simulink model "BattTest"  (Simulink 4.00)
settings: Solver=ode5  StartTime=0.0  StopTime=1  FixedStep=0.01  RelTol=1e-3
values from neighbouring files (symbols this model uses):
  SOC_beg = 70    [AGM_ini_file.m]    (also in DP_Batt_Init.m = battery.init_SOC)
undefined symbols (not defined in the file or in its folder): battery
libraries: simulink3 x6
settings Model: LastModifiedBy=Mark

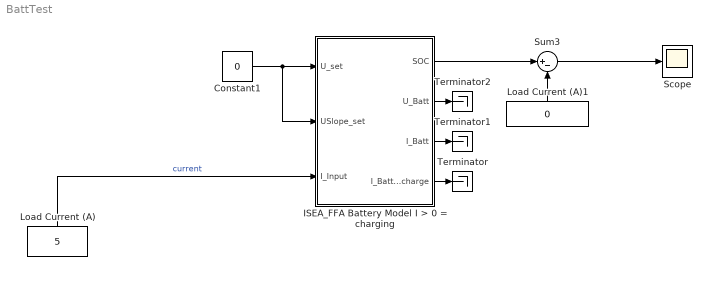
== system BattTest ==
  Constant1 : Constant  Value=0
  ISEA_FFA Battery Model I > 0 = charging : Subsystem
      settings: RTWFcnNameOpts=Auto  RTWFileNameOpts=Auto
  Load Current (A) : Constant  Orientation=up  Value=5
  Load Current (A)1 : Constant  Orientation=up  Value=0
  Scope : Scope
      settings: TimeRange=auto  YMin=-5  YMax=5  SaveToWorkspace=off  SaveName=ScopeData  LimitDataPoints=on  MaxDataPoints=5000
  Sum3 : Sum  Inputs=|+-  SaturateOnIntegerOverflow=on
  Terminator : Terminator
  Terminator1 : Terminator
  Terminator2 : Terminator
  wires:
  Sum3/1 -> Scope/1
  Load Current (A)1/1 -> Sum3/2
  Constant1/1 -> ISEA_FFA Battery Model I > 0 = charging/1(U_set), ISEA_FFA Battery Model I > 0 = charging/2(USlope_set)
  ISEA_FFA Battery Model I > 0 = charging/1(SOC) -> Sum3/1
  ISEA_FFA Battery Model I > 0 = charging/2(U_Batt) -> Terminator2/1
  ISEA_FFA Battery Model I > 0 = charging/3(I_Batt) -> Terminator1/1
  ISEA_FFA Battery Model I > 0 = charging/4(I_Batt_max_charge) -> Terminator/1
  Load Current (A)/1 -> ISEA_FFA Battery Model I > 0 = charging/3(I_Input)  "current"

== system BattTest/ISEA_FFA Battery Model I > 0 = charging ==
  U_set : Inport  Port=1  LatchInput=off
  USlope_set : Inport  Port=2  LatchInput=off
  I_Input : Inport  Port=3  LatchInput=off
  Batterie : Subsystem
      settings: RTWFcnNameOpts=Auto  RTWFileNameOpts=Auto
  Mux : Mux  Inputs=2
  initial battery SOC : Constant  Value=SOC_beg
  SOC : Outport  Port=1
  U_Batt : Outport  Port=2
  I_Batt : Outport  Port=3
  I_Batt_max_charge : Outport  Port=4
  wires:
  Batterie/4(SOC) -> SOC/1
  Batterie/3(BUS_U_out) -> U_Batt/1  "BUS_U"
  Mux/1 -> Batterie/1(BUS_1_in1)  "BUS_1"
  initial battery SOC/1 -> Mux/2  "SOC_beg"
  I_Input/1 -> Mux/1
  Batterie/2(I_Batt) -> I_Batt/1
  U_set/1 -> Batterie/2(U_set)
  Batterie/1(I_Batt_max_charge) -> I_Batt_max_charge/1
  USlope_set/1 -> Batterie/3(USlope_set)

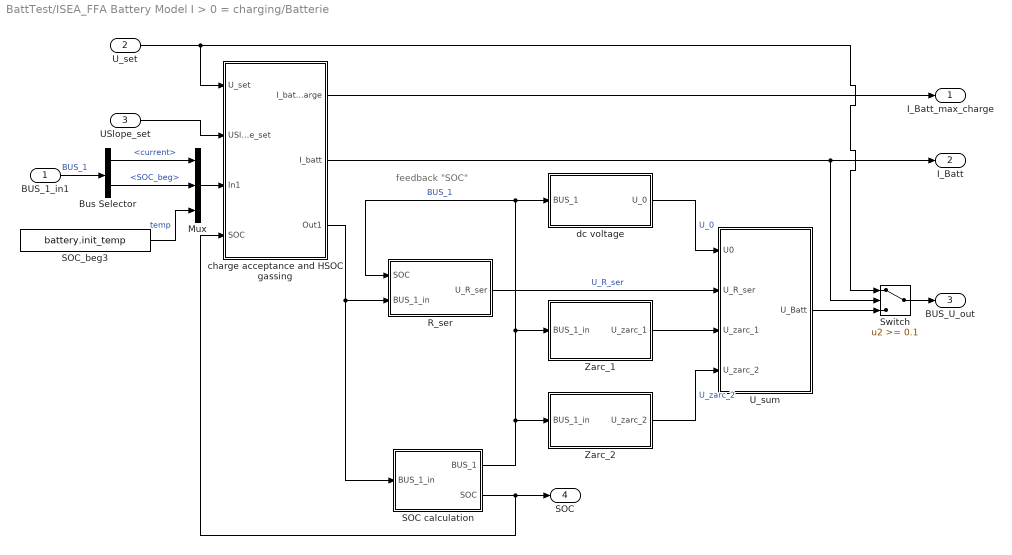
== system BattTest/ISEA_FFA Battery Model I > 0 = charging/Batterie ==
  note: feedback "SOC"
  BUS_1_in1 : Inport  Port=1  LatchInput=off
  U_set : Inport  Port=2  LatchInput=off
  USlope_set : Inport  Port=3  LatchInput=off
  Bus Selector : BusSelector  OutputSignals=current,SOC_beg  MuxedOutput=off
  Mux : Mux  Inputs=3
  R_ser : Subsystem
      settings: RTWFcnNameOpts=Auto  RTWFileNameOpts=Auto
  SOC calculation : Subsystem
      settings: RTWFcnNameOpts=Auto  RTWFileNameOpts=Auto
  SOC_beg3 : Constant  Value=battery.init_temp
  Switch : Switch  Threshold=0.1
  U_sum : Subsystem
      settings: RTWFcnNameOpts=Auto  RTWFileNameOpts=Auto
  Zarc_1 : Subsystem
      settings: RTWFcnNameOpts=Auto  RTWFileNameOpts=Auto
  Zarc_2 : Subsystem
      settings: RTWFcnNameOpts=Auto  RTWFileNameOpts=Auto
  charge acceptance and HSOC gassing : Subsystem
      settings: RTWFcnNameOpts=Auto  RTWFileNameOpts=Auto
  dc voltage : Subsystem
      settings: RTWFcnNameOpts=Auto  RTWFileNameOpts=Auto
  I_Batt_max_charge : Outport  Port=1
  I_Batt : Outport  Port=2
  BUS_U_out : Outport  Port=3
  SOC : Outport  Port=4
  wires:
  SOC calculation/2(SOC) -> SOC/1, charge acceptance and HSOC gassing/4(SOC)
  SOC_beg3/1 -> Mux/3  "temp"
  BUS_1_in1/1 -> Bus Selector/1  "BUS_1"
  Mux/1 -> charge acceptance and HSOC gassing/3(In1)
  Bus Selector/2 -> Mux/2  "<SOC_beg>"
  Bus Selector/1 -> Mux/1  "<current>"
  Zarc_1/1(U_zarc_1) -> U_sum/3(U_zarc_1)
  Zarc_2/1(U_zarc_2) -> U_sum/4(U_zarc_2)  "U_zarc_2"
  SOC calculation/1(BUS_1) -> Zarc_2/1(BUS_1_in), dc voltage/1(BUS_1), R_ser/1(SOC), Zarc_1/1(BUS_1_in)  "BUS_1"
  dc voltage/1(U_0) -> U_sum/1(U0)  "U_0"
  R_ser/1(U_R_ser) -> U_sum/2(U_R_ser)  "U_R_ser"
  charge acceptance and HSOC gassing/3(Out1) -> R_ser/2(BUS_1_in), SOC calculation/1(BUS_1_in)
  U_sum/1(U_Batt) -> Switch/3
  Switch/1 -> BUS_U_out/1
  charge acceptance and HSOC gassing/2(I_batt) -> I_Batt/1, Switch/2
  charge acceptance and HSOC gassing/1(I_bat_max_charge) -> I_Batt_max_charge/1
  USlope_set/1 -> charge acceptance and HSOC gassing/2(USlope_set)
  U_set/1 -> charge acceptance and HSOC gassing/1(U_set), Switch/1

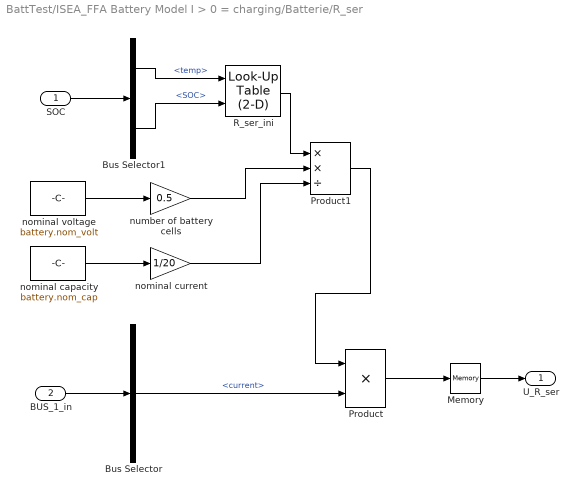
== system BattTest/ISEA_FFA Battery Model I > 0 = charging/Batterie/R_ser ==
  SOC : Inport  Port=1  LatchInput=off
  BUS_1_in : Inport  Port=2  LatchInput=off
  Bus Selector : BusSelector  OutputSignals=current  MuxedOutput=off
  Bus Selector1 : BusSelector  OutputSignals=temp,SOC  MuxedOutput=off
  Memory : Memory  X0=0  InheritSampleTime=off
      settings: RTWStateStorageClass=Auto
  Product : Product  Inputs=2  Multiplication=Element-wise(.*)  SaturateOnIntegerOverflow=on
  Product1 : Product  Inputs=**/  Multiplication=Element-wise(.*)  SaturateOnIntegerOverflow=on
  R_ser_ini : simulink3/Functions & Tables/Look-Up Table (2-D)  x=battery.temp_in  y=battery.SOC_in  t=battery.R_ser_ini
  nominal capacity : Constant  Value=battery.nom_cap
  nominal current : Gain  Gain=1/20  Multiplication=Element-wise(K.*u)  SaturateOnIntegerOverflow=on
  nominal voltage : Constant  Value=battery.nom_volt
  number of battery cells : Gain  Gain=0.5  Multiplication=Element-wise(K.*u)  SaturateOnIntegerOverflow=on
  U_R_ser : Outport  Port=1
  wires:
  Memory/1 -> U_R_ser/1
  nominal capacity/1 -> nominal current/1
  nominal current/1 -> Product1/3
  Product1/1 -> Product/1
  number of battery cells/1 -> Product1/2
  nominal voltage/1 -> number of battery cells/1
  R_ser_ini/1 -> Product1/1
  Bus Selector1/1 -> R_ser_ini/1  "<temp>"
  Bus Selector1/2 -> R_ser_ini/2  "<SOC>"
  SOC/1 -> Bus Selector1/1
  Product/1 -> Memory/1
  Bus Selector/1 -> Product/2  "<current>"
  BUS_1_in/1 -> Bus Selector/1

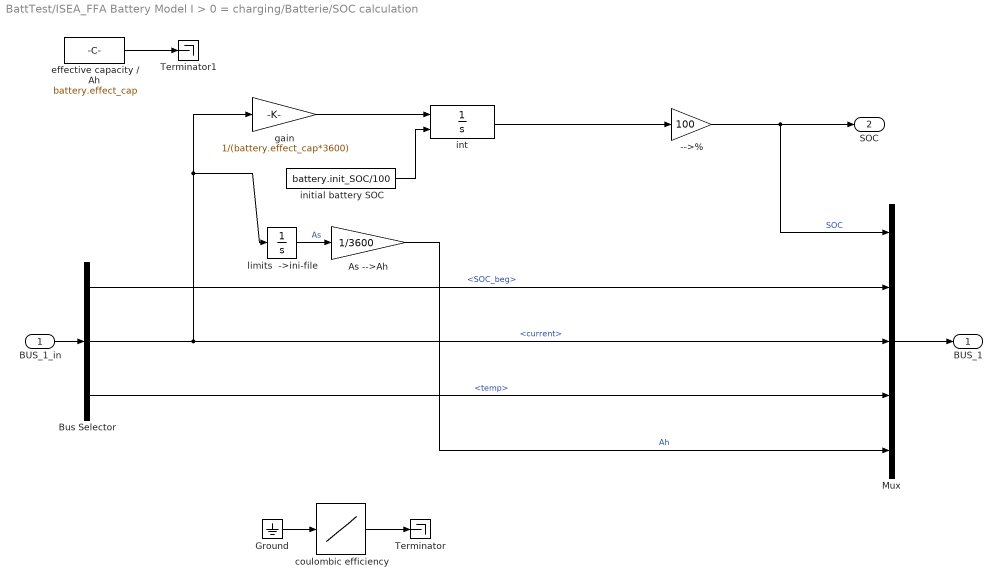
== system BattTest/ISEA_FFA Battery Model I > 0 = charging/Batterie/SOC calculation ==
  BUS_1_in : Inport  Port=1  LatchInput=off
  -->% : Gain  Gain=100  Multiplication=Element-wise(K.*u)  SaturateOnIntegerOverflow=on
  As -->Ah : Gain  Gain=1/3600  Multiplication=Element-wise(K.*u)  SaturateOnIntegerOverflow=on
  Bus Selector : BusSelector  OutputSignals=SOC_beg,current,temp  MuxedOutput=off
  Ground : Ground
  Mux : Mux  Inputs=5
  Terminator : Terminator
  Terminator1 : Terminator
  coulombic efficiency : Lookup  InputValues=[-1 0 1]  OutputValues=[-1 0 battery.eta_coulomb/100]
  "effective capacity / Ah " : Constant  Value=battery.effect_cap
  gain : Gain  Gain=1/(battery.effect_cap*3600)  Multiplication=Element-wise(K.*u)  SaturateOnIntegerOverflow=on
  initial battery SOC : Constant  Value=battery.init_SOC/100
  int : Integrator  ExternalReset=none  InitialConditionSource=external  InitialCondition=0  LimitOutput=on  UpperSaturationLimit=1  LowerSaturationLimit=0  ShowSaturationPort=off  ShowStatePort=off  AbsoluteTolerance=auto
  limits  ->ini-file : Integrator  ExternalReset=none  InitialConditionSource=internal  InitialCondition=0  LimitOutput=on  UpperSaturationLimit=battery.up_lim_soc_calc  LowerSaturationLimit=battery.low_lim_soc_calc  ShowSaturationPort=off  ShowStatePort=off  AbsoluteTolerance=auto
  BUS_1 : Outport  Port=1
  SOC : Outport  Port=2
  wires:
  -->%/1 -> Mux/1, SOC/1  "SOC"
  int/1 -> -->%/1
  As -->Ah/1 -> Mux/5  "Ah"
  limits  ->ini-file/1 -> As -->Ah/1  "As"
  Bus Selector/1 -> Mux/2  "<SOC_beg>"
  Bus Selector/2 -> Mux/3, limits  ->ini-file/1, gain/1  "<current>"
  Mux/1 -> BUS_1/1
  Bus Selector/3 -> Mux/4  "<temp>"
  BUS_1_in/1 -> Bus Selector/1
  Ground/1 -> coulombic efficiency/1
  coulombic efficiency/1 -> Terminator/1
  initial battery SOC/1 -> int/2
  gain/1 -> int/1
  "effective capacity / Ah "/1 -> Terminator1/1

== system BattTest/ISEA_FFA Battery Model I > 0 = charging/Batterie/U_sum ==
  U0 : Inport  Port=1  LatchInput=off
  U_R_ser : Inport  Port=2  LatchInput=off
  U_zarc_1 : Inport  Port=3  LatchInput=off
  U_zarc_2 : Inport  Port=4  LatchInput=off
  Bus Selector2 : BusSelector  OutputSignals=U_2c,U_2b,U_2d  MuxedOutput=off
  Sum : Sum  Inputs=+++++  SaturateOnIntegerOverflow=on
  Sum3 : Sum  Inputs=+++  SaturateOnIntegerOverflow=on
  U_L : Constant  Value=0
  U_Batt : Outport  Port=1
  wires:
  U_L/1 -> Sum/2
  U_zarc_1/1 -> Sum/4
  U_zarc_2/1 -> Bus Selector2/1
  Sum3/1 -> Sum/5
  U0/1 -> Sum/1
  Bus Selector2/3 -> Sum3/3  "<U_2d>"
  Bus Selector2/2 -> Sum3/2  "<U_2b>"
  Bus Selector2/1 -> Sum3/1  "<U_2c>"
  Sum/1 -> U_Batt/1  "U_ges"
  U_R_ser/1 -> Sum/3

== system BattTest/ISEA_FFA Battery Model I > 0 = charging/Batterie/Zarc_1 ==
  BUS_1_in : Inport  Port=1  LatchInput=off
  Bus Selector : BusSelector  OutputSignals=current  MuxedOutput=off
  Look-Up for 60 Ah vlies tec : Lookup  InputValues=battery.zarc1_linearity(:,1)  OutputValues=battery.zarc1_linearity(:,2)
  Model Info : simulink3/Signals & Systems/Model Info  InitialBlockCM=None  BlockCM=None  Frame=on  DisplayStringWithTags=|  HorizontalTextAlignment=Center  LeftAlignmentValue=0.5  SourceBlockDiagram=BattTest  TagMaxNumber=20
      | Model Info
      | %<ModifiedBy>
      | %<ModifiedDate>
      | %<Description>
      | sploumen: deleted isea's original ZARC_1 voltage calculation, since it has static behaviour that can\n be described using 1-D look-up as function of current.
  Product3 : Product  Inputs=**/  Multiplication=Element-wise(.*)  SaturateOnIntegerOverflow=on
  lookup table is for 60 Ah : Constant  Value=60
  nominal capacity : Constant  Value=battery.nom_cap
  U_zarc_1 : Outport  Port=1
  wires:
  Product3/1 -> U_zarc_1/1  "U_zarc1"
  nominal capacity/1 -> Product3/3
  BUS_1_in/1 -> Bus Selector/1  "BUS_1"
  Bus Selector/1 -> Look-Up for 60 Ah vlies tec/1  "<current>"
  lookup table is for 60 Ah/1 -> Product3/2
  Look-Up for 60 Ah vlies tec/1 -> Product3/1

== system BattTest/ISEA_FFA Battery Model I > 0 = charging/Batterie/Zarc_2 ==
  note: BUS_1:  <charge current>
      |           <SOC>
      |            <temp>
  BUS_1_in : Inport  Port=1  LatchInput=off
  Bus Selector1 : BusSelector  OutputSignals=temp,SOC  MuxedOutput=off
  C_2eff_ini : simulink3/Functions & Tables/Look-Up Table (2-D)  x=battery.temp_in  y=battery.SOC_in  t=battery.C_2eff_ini
  "Freq1_3 " : Lookup  InputValues=battery.phi_in  OutputValues=battery.Freq1_3
  I_0_ini : simulink3/Functions & Tables/Look-Up Table (2-D)  x=battery.temp_in  y=battery.SOC_in  t=battery.I_0_ini
  Mux : Mux  Inputs=5
  RC_Glied_2b : Subsystem
      settings: RTWFcnNameOpts=Auto  RTWFileNameOpts=Auto
  RC_Glied_2c : Subsystem
      settings: RTWFcnNameOpts=Auto  RTWFileNameOpts=Auto
  RC_Glied_2d : Subsystem
      settings: RTWFcnNameOpts=Auto  RTWFileNameOpts=Auto
  alpha : simulink3/Functions & Tables/Look-Up Table (2-D)  x=battery.temp_in  y=battery.SOC_in  t=battery.alpha
  calculation U_T : Subsystem
      settings: RTWFcnNameOpts=Auto  RTWFileNameOpts=Auto
  phi_2 : simulink3/Functions & Tables/Look-Up Table (2-D)  x=battery.temp_in  y=battery.SOC_in  t=battery.phi_2
  U_zarc_2 : Outport  Port=1
  wires:
  I_0_ini/1 -> Mux/3  "I_0_ini"
  C_2eff_ini/1 -> Mux/4  "C_2eff/IN"
  RC_Glied_2d/1(BUS_2_out) -> U_zarc_2/1
  Mux/1 -> RC_Glied_2c/2(Para_Bus)
  "Freq1_3 "/1 -> Mux/5  "Freq1_3"
  alpha/1 -> Mux/2  "alpha"
  calculation U_T/1(U_T) -> Mux/1  "U_T"
  phi_2/1 -> "Freq1_3 "/1
  Bus Selector1/1 -> phi_2/1, C_2eff_ini/1, I_0_ini/1, calculation U_T/1(temp), alpha/1  "<temp>"
  Bus Selector1/2 -> phi_2/2, C_2eff_ini/2, I_0_ini/2, alpha/2  "<SOC>"
  RC_Glied_2b/1(BUS_2_out) -> RC_Glied_2d/1(BUS_2_in)
  RC_Glied_2c/1(BUS_2_out) -> RC_Glied_2b/1(BUS_2_in)
  BUS_1_in/1 -> Bus Selector1/1, RC_Glied_2c/1(BUS_1_in), RC_Glied_2d/2(BUS_1_in), RC_Glied_2b/2(BUS_1_in)

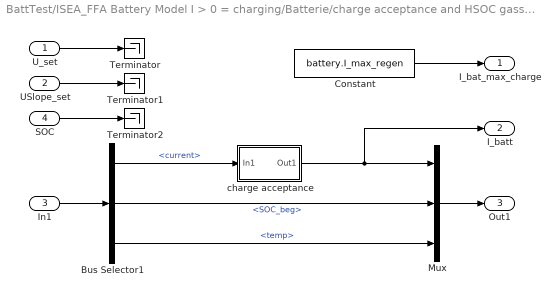
== system BattTest/ISEA_FFA Battery Model I > 0 = charging/Batterie/charge acceptance and HSOC gassing ==
  U_set : Inport  Port=1  LatchInput=off
  USlope_set : Inport  Port=2  LatchInput=off
  In1 : Inport  Port=3  LatchInput=off
  SOC : Inport  Port=4  LatchInput=off
  Bus Selector1 : BusSelector  OutputSignals=current,SOC_beg,temp  MuxedOutput=off
  Constant : Constant  Value=battery.I_max_regen
  Mux : Mux  Inputs=3
  Terminator : Terminator
  Terminator1 : Terminator
  Terminator2 : Terminator
  charge acceptance : Subsystem
      settings: RTWFcnNameOpts=Auto  RTWFileNameOpts=Auto
  I_bat_max_charge : Outport  Port=1
  I_batt : Outport  Port=2
  Out1 : Outport  Port=3
  wires:
  In1/1 -> Bus Selector1/1
  Bus Selector1/2 -> Mux/2  "<SOC_beg>"
  Bus Selector1/3 -> Mux/3  "<temp>"
  Mux/1 -> Out1/1
  Bus Selector1/1 -> charge acceptance/1(In1)  "<current>"
  charge acceptance/1(Out1) -> Mux/1, I_batt/1
  U_set/1 -> Terminator/1
  USlope_set/1 -> Terminator1/1
  SOC/1 -> Terminator2/1
  Constant/1 -> I_bat_max_charge/1

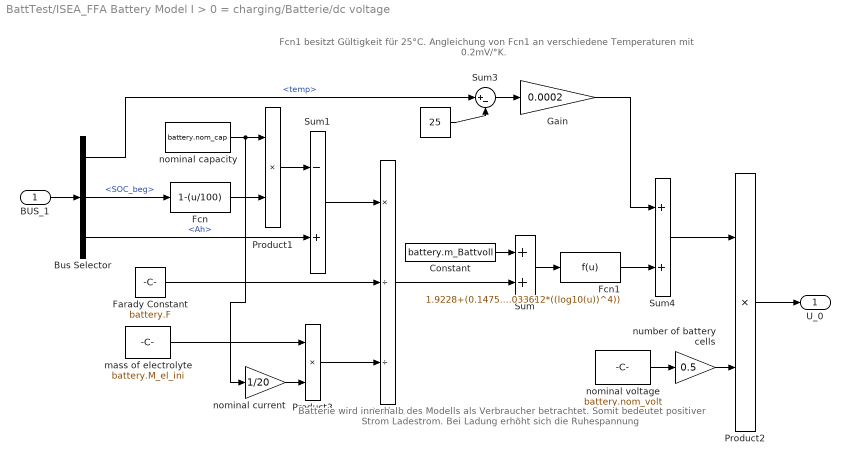
== system BattTest/ISEA_FFA Battery Model I > 0 = charging/Batterie/dc voltage ==
  note: Fcn1 besitzt Gültigkeit für 25°C.
      | Angleichung von Fcn1 an verschiedene
      | Temperaturen mit 0.2mV/°K.
  note: Batterie wird innerhalb des
      | Modells als Verbraucher
      | betrachtet. Somit bedeutet
      | positiver Strom Ladestrom.
      | Bei Ladung erhöht sich die
      | Ruhespannung
  BUS_1 : Inport  Port=1  LatchInput=off
  " " : Constant  Value=25
  Bus Selector : BusSelector  OutputSignals=temp,SOC_beg,Ah  MuxedOutput=off
  Constant : Constant  Value=battery.m_Battvoll
  Farady Constant : Constant  Value=battery.F
  Fcn : Fcn  Expr=1-(u/100)
  Fcn1 : Fcn  Expr=1.9228+(0.147519*(log10(u)))+(0.063552*((log10(u))^2))+(0.073772*((log10(u))^3))+(0.033612*((log10(u))^4))
  Gain : Gain  Gain=0.0002  Multiplication=Element-wise(K.*u)  SaturateOnIntegerOverflow=on
  Product : Product  Inputs=*//  Multiplication=Element-wise(.*)  SaturateOnIntegerOverflow=on
  Product1 : Product  Inputs=**  Multiplication=Element-wise(.*)  SaturateOnIntegerOverflow=on
  Product2 : Product  Inputs=**  Multiplication=Element-wise(.*)  SaturateOnIntegerOverflow=on
  Product3 : Product  Inputs=**  Multiplication=Element-wise(.*)  SaturateOnIntegerOverflow=on
  Sum : Sum  Inputs=++  SaturateOnIntegerOverflow=on
  Sum1 : Sum  Inputs=-+  SaturateOnIntegerOverflow=on
  Sum3 : Sum  Inputs=|+-  SaturateOnIntegerOverflow=on
  Sum4 : Sum  Inputs=++  SaturateOnIntegerOverflow=on
  mass of electrolyte : Constant  Value=battery.M_el_ini
  nominal capacity : Constant  Value=battery.nom_cap
  nominal current : Gain  Gain=1/20  Multiplication=Element-wise(K.*u)  SaturateOnIntegerOverflow=on
  nominal voltage : Constant  Value=battery.nom_volt
  number of battery cells : Gain  Gain=0.5  Multiplication=Element-wise(K.*u)  SaturateOnIntegerOverflow=on
  U_0 : Outport  Port=1
  wires:
  nominal current/1 -> Product3/2
  mass of electrolyte/1 -> Product3/1
  Product3/1 -> Product/3
  number of battery cells/1 -> Product2/2
  nominal voltage/1 -> number of battery cells/1
  Gain/1 -> Sum4/1
  Sum4/1 -> Product2/1
  Sum3/1 -> Gain/1
  " "/1 -> Sum3/2
  Bus Selector/1 -> Sum3/1  "<temp>"
  Product2/1 -> U_0/1
  Fcn1/1 -> Sum4/2
  Sum1/1 -> Product/1
  Bus Selector/3 -> Sum1/2  "<Ah>"
  Product1/1 -> Sum1/1
  Fcn/1 -> Product1/2
  Bus Selector/2 -> Fcn/1  "<SOC_beg>"
  nominal capacity/1 -> nominal current/1, Product1/1
  Sum/1 -> Fcn1/1
  Constant/1 -> Sum/1
  Product/1 -> Sum/2
  Farady Constant/1 -> Product/2
  BUS_1/1 -> Bus Selector/1

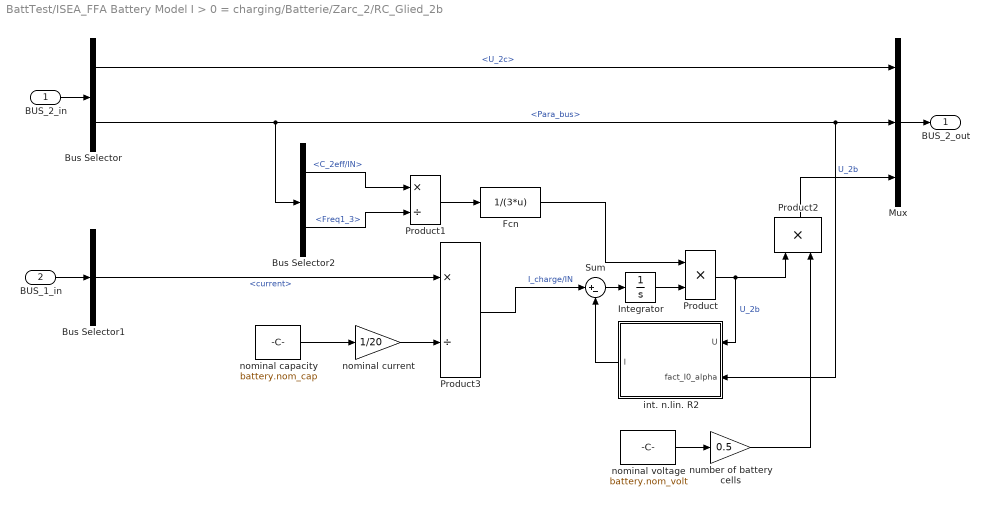
== system BattTest/ISEA_FFA Battery Model I > 0 = charging/Batterie/Zarc_2/RC_Glied_2b ==
  BUS_2_in : Inport  Port=1  LatchInput=off
  BUS_1_in : Inport  Port=2  LatchInput=off
  Bus Selector : BusSelector  OutputSignals=U_2c,Para_bus  MuxedOutput=off
  Bus Selector1 : BusSelector  OutputSignals=current  MuxedOutput=off
  Bus Selector2 : BusSelector  OutputSignals=C_2eff/IN,Freq1_3  MuxedOutput=off
  Fcn : Fcn  Expr=1/(3*u)
  Integrator : Integrator  ExternalReset=none  InitialConditionSource=internal  InitialCondition=0.1  LimitOutput=off  UpperSaturationLimit=inf  LowerSaturationLimit=-inf  ShowSaturationPort=off  ShowStatePort=off  AbsoluteTolerance=auto
  Mux : Mux  Inputs=3
  Product : Product  Inputs=2  Multiplication=Element-wise(.*)  SaturateOnIntegerOverflow=on
  Product1 : Product  Inputs=*/  Multiplication=Element-wise(.*)  SaturateOnIntegerOverflow=on
  Product2 : Product  Orientation=up  Inputs=2  Multiplication=Element-wise(.*)  SaturateOnIntegerOverflow=on
  Product3 : Product  Inputs=*/  Multiplication=Element-wise(.*)  SaturateOnIntegerOverflow=on
  Sum : Sum  Inputs=|+-  SaturateOnIntegerOverflow=on
  int. n.lin. R2 : Subsystem  Orientation=left
      settings: RTWFcnNameOpts=Auto  RTWFileNameOpts=Auto
  nominal capacity : Constant  Value=battery.nom_cap
  nominal current : Gain  Gain=1/20  Multiplication=Element-wise(K.*u)  SaturateOnIntegerOverflow=on
  nominal voltage : Constant  Value=battery.nom_volt
  number of battery cells : Gain  Gain=0.5  Multiplication=Element-wise(K.*u)  SaturateOnIntegerOverflow=on
  BUS_2_out : Outport  Port=1
  wires:
  Bus Selector1/1 -> Product3/1  "<current>"
  nominal current/1 -> Product3/2
  nominal capacity/1 -> nominal current/1
  Product3/1 -> Sum/1  "I_charge/IN"
  number of battery cells/1 -> Product2/2
  nominal voltage/1 -> number of battery cells/1
  Fcn/1 -> Product/1
  Product1/1 -> Fcn/1
  Bus Selector2/2 -> Product1/2  "<Freq1_3>"
  Bus Selector2/1 -> Product1/1  "<C_2eff/IN>"
  Bus Selector/2 -> Bus Selector2/1, Mux/2, int. n.lin. R2/2(fact_I0_alpha)  "<Para_bus>"
  Bus Selector/1 -> Mux/1  "<U_2c>"
  Product2/1 -> Mux/3  "U_2b"
  Mux/1 -> BUS_2_out/1
  BUS_1_in/1 -> Bus Selector1/1
  Product/1 -> Product2/1, int. n.lin. R2/1(U)  "U_2b"
  int. n.lin. R2/1(I) -> Sum/2
  Sum/1 -> Integrator/1
  Integrator/1 -> Product/2
  BUS_2_in/1 -> Bus Selector/1

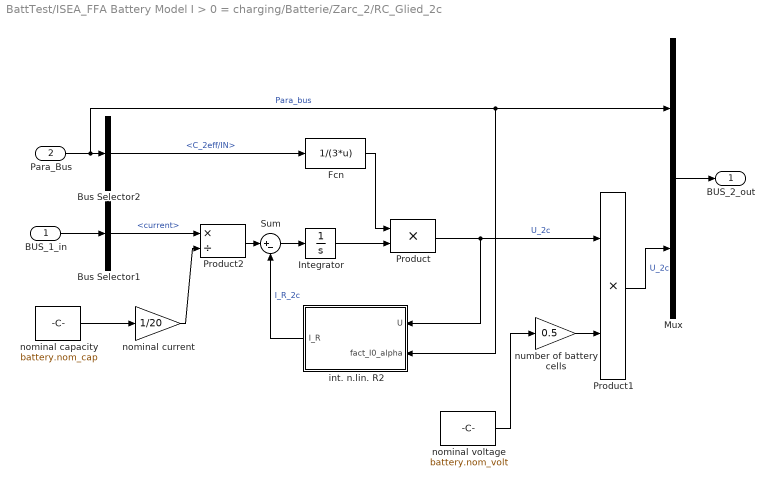
== system BattTest/ISEA_FFA Battery Model I > 0 = charging/Batterie/Zarc_2/RC_Glied_2c ==
  BUS_1_in : Inport  Port=1  LatchInput=off
  Para_Bus : Inport  Port=2  LatchInput=off
  Bus Selector1 : BusSelector  OutputSignals=current  MuxedOutput=off
  Bus Selector2 : BusSelector  OutputSignals=C_2eff/IN  MuxedOutput=off
  Fcn : Fcn  Expr=1/(3*u)
  Integrator : Integrator  ExternalReset=none  InitialConditionSource=internal  InitialCondition=0.1  LimitOutput=off  UpperSaturationLimit=inf  LowerSaturationLimit=-inf  ShowSaturationPort=off  ShowStatePort=off  AbsoluteTolerance=auto
  Mux : Mux  Inputs=2
  Product : Product  Inputs=2  Multiplication=Element-wise(.*)  SaturateOnIntegerOverflow=on
  Product1 : Product  Inputs=2  Multiplication=Element-wise(.*)  SaturateOnIntegerOverflow=on
  Product2 : Product  Inputs=*/  Multiplication=Element-wise(.*)  SaturateOnIntegerOverflow=on
  Sum : Sum  Inputs=|+-  SaturateOnIntegerOverflow=on
  int. n.lin. R2 : Subsystem  Orientation=left
      settings: RTWFcnNameOpts=Auto  RTWFileNameOpts=Auto
  nominal capacity : Constant  Value=battery.nom_cap
  nominal current : Gain  Gain=1/20  Multiplication=Element-wise(K.*u)  SaturateOnIntegerOverflow=on
  nominal voltage : Constant  Value=battery.nom_volt
  number of battery cells : Gain  Gain=0.5  Multiplication=Element-wise(K.*u)  SaturateOnIntegerOverflow=on
  BUS_2_out : Outport  Port=1
  wires:
  nominal current/1 -> Product2/2
  Bus Selector1/1 -> Product2/1  "<current>"
  Product2/1 -> Sum/1
  nominal capacity/1 -> nominal current/1
  number of battery cells/1 -> Product1/2
  nominal voltage/1 -> number of battery cells/1
  Mux/1 -> BUS_2_out/1
  Fcn/1 -> Product/1
  Bus Selector2/1 -> Fcn/1  "<C_2eff/IN>"
  Para_Bus/1 -> Mux/1, int. n.lin. R2/2(fact_I0_alpha), Bus Selector2/1  "Para_bus"
  Product1/1 -> Mux/2  "U_2c"
  int. n.lin. R2/1(I_R) -> Sum/2  "I_R_2c"
  BUS_1_in/1 -> Bus Selector1/1
  Sum/1 -> Integrator/1
  Product/1 -> Product1/1, int. n.lin. R2/1(U)  "U_2c"
  Integrator/1 -> Product/2

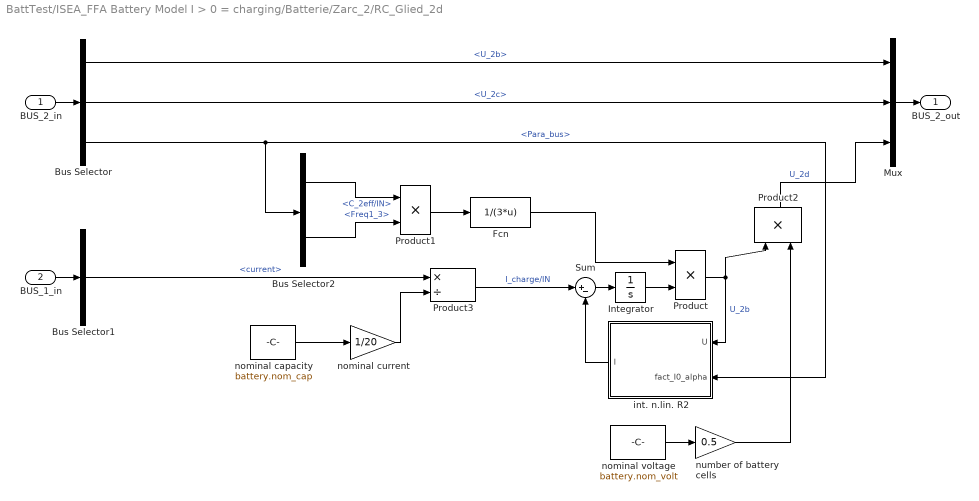
== system BattTest/ISEA_FFA Battery Model I > 0 = charging/Batterie/Zarc_2/RC_Glied_2d ==
  BUS_2_in : Inport  Port=1  LatchInput=off
  BUS_1_in : Inport  Port=2  LatchInput=off
  Bus Selector : BusSelector  OutputSignals=U_2b,U_2c,Para_bus  MuxedOutput=off
  Bus Selector1 : BusSelector  OutputSignals=current  MuxedOutput=off
  Bus Selector2 : BusSelector  OutputSignals=C_2eff/IN,Freq1_3  MuxedOutput=off
  Fcn : Fcn  Expr=1/(3*u)
  Integrator : Integrator  ExternalReset=none  InitialConditionSource=internal  InitialCondition=0.1  LimitOutput=off  UpperSaturationLimit=inf  LowerSaturationLimit=-inf  ShowSaturationPort=off  ShowStatePort=off  AbsoluteTolerance=auto
  Mux : Mux  Inputs=3
  Product : Product  Inputs=2  Multiplication=Element-wise(.*)  SaturateOnIntegerOverflow=on
  Product1 : Product  Inputs=**  Multiplication=Element-wise(.*)  SaturateOnIntegerOverflow=on
  Product2 : Product  Orientation=up  Inputs=2  Multiplication=Element-wise(.*)  SaturateOnIntegerOverflow=on
  Product3 : Product  Inputs=*/  Multiplication=Element-wise(.*)  SaturateOnIntegerOverflow=on
  Sum : Sum  Inputs=|+-  SaturateOnIntegerOverflow=on
  int. n.lin. R2 : Subsystem  Orientation=left
      settings: RTWFcnNameOpts=Auto  RTWFileNameOpts=Auto
  nominal capacity : Constant  Value=battery.nom_cap
  nominal current : Gain  Gain=1/20  Multiplication=Element-wise(K.*u)  SaturateOnIntegerOverflow=on
  nominal voltage : Constant  Value=battery.nom_volt
  number of battery cells : Gain  Gain=0.5  Multiplication=Element-wise(K.*u)  SaturateOnIntegerOverflow=on
  BUS_2_out : Outport  Port=1
  wires:
  Bus Selector1/1 -> Product3/1  "<current>"
  Product3/1 -> Sum/1  "I_charge/IN"
  nominal current/1 -> Product3/2
  nominal capacity/1 -> nominal current/1
  number of battery cells/1 -> Product2/2
  nominal voltage/1 -> number of battery cells/1
  Bus Selector/2 -> Mux/2  "<U_2c>"
  Bus Selector/1 -> Mux/1  "<U_2b>"
  Product2/1 -> Mux/3  "U_2d"
  Fcn/1 -> Product/1
  Product1/1 -> Fcn/1
  Bus Selector2/2 -> Product1/2  "<Freq1_3>"
  Bus Selector2/1 -> Product1/1  "<C_2eff/IN>"
  Bus Selector/3 -> int. n.lin. R2/2(fact_I0_alpha), Bus Selector2/1  "<Para_bus>"
  Mux/1 -> BUS_2_out/1
  BUS_1_in/1 -> Bus Selector1/1
  Product/1 -> Product2/1, int. n.lin. R2/1(U)  "U_2b"
  int. n.lin. R2/1(I) -> Sum/2
  Sum/1 -> Integrator/1
  Integrator/1 -> Product/2
  BUS_2_in/1 -> Bus Selector/1

== system BattTest/ISEA_FFA Battery Model I > 0 = charging/Batterie/Zarc_2/calculation U_T ==
  note: °C -> °K
  temp : Inport  Port=1  LatchInput=off
  Ah .. As : Gain  Gain=3600  Multiplication=Element-wise(K.*u)  SaturateOnIntegerOverflow=on
  Constant : Constant  Value=273.15
  Constant1 : Constant  Value=battery.R
  Constant2 : Constant  Value=battery.F
  Product : Product  Inputs=**/  Multiplication=Element-wise(.*)  SaturateOnIntegerOverflow=on
  Sum : Sum  Inputs=++  SaturateOnIntegerOverflow=on
  U_T : Outport  Port=1
  wires:
  Product/1 -> U_T/1
  Ah .. As/1 -> Product/3
  Constant2/1 -> Ah .. As/1
  Constant1/1 -> Product/2
  Sum/1 -> Product/1
  temp/1 -> Sum/2
  Constant/1 -> Sum/1

== system BattTest/ISEA_FFA Battery Model I > 0 = charging/Batterie/charge acceptance and HSOC gassing/charge acceptance ==
  In1 : Inport  Port=1  LatchInput=off
  Out1 : Outport  Port=1
  wires:
  In1/1 -> Out1/1

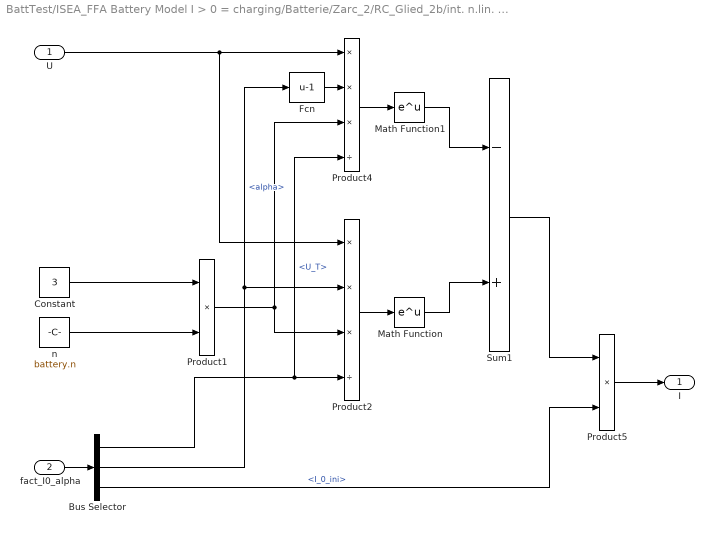
== system BattTest/ISEA_FFA Battery Model I > 0 = charging/Batterie/Zarc_2/RC_Glied_2b/int. n.lin. R2 ==
  U : Inport  Port=1  LatchInput=off
  fact_I0_alpha : Inport  Port=2  LatchInput=off
  Bus Selector : BusSelector  OutputSignals=U_T,alpha,I_0_ini  MuxedOutput=off
  Constant : Constant  Value=3
  Fcn : Fcn  Expr=u-1
  Math Function : Math  Operator=exp  OutputSignalType=auto
  Math Function1 : Math  Operator=exp  OutputSignalType=auto
  Product1 : Product  Inputs=**  Multiplication=Element-wise(.*)  SaturateOnIntegerOverflow=on
  Product2 : Product  Inputs=***/  Multiplication=Element-wise(.*)  SaturateOnIntegerOverflow=on
  Product4 : Product  Inputs=***/  Multiplication=Element-wise(.*)  SaturateOnIntegerOverflow=on
  Product5 : Product  Inputs=**  Multiplication=Element-wise(.*)  SaturateOnIntegerOverflow=on
  Sum1 : Sum  Inputs=-+  SaturateOnIntegerOverflow=on
  n : Constant  Value=battery.n
  I : Outport  Port=1
  wires:
  Constant/1 -> Product1/1
  Bus Selector/3 -> Product5/2  "<I_0_ini>"
  Product1/1 -> Product4/3, Product2/3
  n/1 -> Product1/2
  Product4/1 -> Math Function1/1
  Product5/1 -> I/1
  Sum1/1 -> Product5/1
  Math Function/1 -> Sum1/2
  Math Function1/1 -> Sum1/1
  Product2/1 -> Math Function/1
  U/1 -> Product2/1, Product4/1
  Fcn/1 -> Product4/2
  Bus Selector/2 -> Fcn/1, Product2/2  "<alpha>"
  Bus Selector/1 -> Product4/4, Product2/4  "<U_T>"
  fact_I0_alpha/1 -> Bus Selector/1

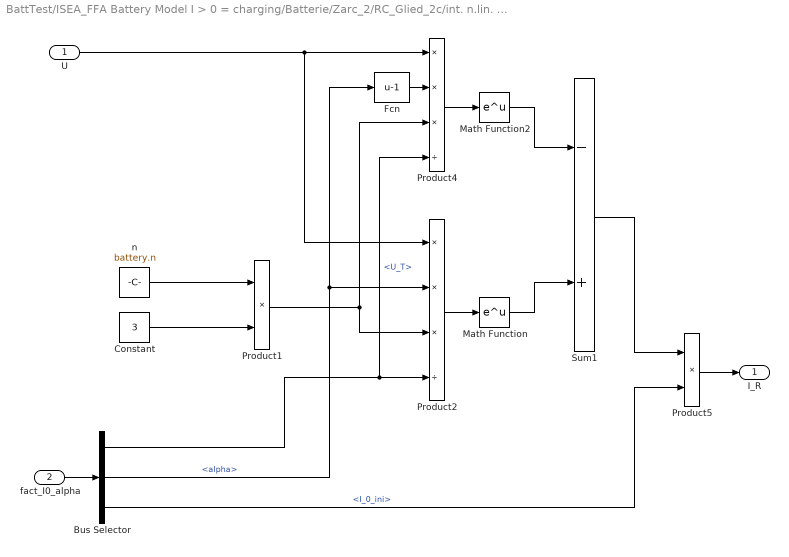
== system BattTest/ISEA_FFA Battery Model I > 0 = charging/Batterie/Zarc_2/RC_Glied_2c/int. n.lin. R2 ==
  U : Inport  Port=1  LatchInput=off
  fact_I0_alpha : Inport  Port=2  LatchInput=off
  Bus Selector : BusSelector  OutputSignals=U_T,alpha,I_0_ini  MuxedOutput=off
  Constant : Constant  Value=3
  Fcn : Fcn  Expr=u-1
  Math Function : Math  Operator=exp  OutputSignalType=auto
  Math Function2 : Math  Operator=exp  OutputSignalType=auto
  Product1 : Product  Inputs=**  Multiplication=Element-wise(.*)  SaturateOnIntegerOverflow=on
  Product2 : Product  Inputs=***/  Multiplication=Element-wise(.*)  SaturateOnIntegerOverflow=on
  Product4 : Product  Inputs=***/  Multiplication=Element-wise(.*)  SaturateOnIntegerOverflow=on
  Product5 : Product  Inputs=**  Multiplication=Element-wise(.*)  SaturateOnIntegerOverflow=on
  Sum1 : Sum  Inputs=-+  SaturateOnIntegerOverflow=on
  n : Constant  Value=battery.n
  I_R : Outport  Port=1
  wires:
  fact_I0_alpha/1 -> Bus Selector/1
  Constant/1 -> Product1/2
  Product1/1 -> Product4/3, Product2/3
  n/1 -> Product1/1
  Product5/1 -> I_R/1
  Sum1/1 -> Product5/1
  Bus Selector/3 -> Product5/2  "<I_0_ini>"
  Math Function/1 -> Sum1/2
  Math Function2/1 -> Sum1/1
  Product4/1 -> Math Function2/1
  Product2/1 -> Math Function/1
  U/1 -> Product2/1, Product4/1
  Fcn/1 -> Product4/2
  Bus Selector/2 -> Fcn/1, Product2/2  "<alpha>"
  Bus Selector/1 -> Product4/4, Product2/4  "<U_T>"

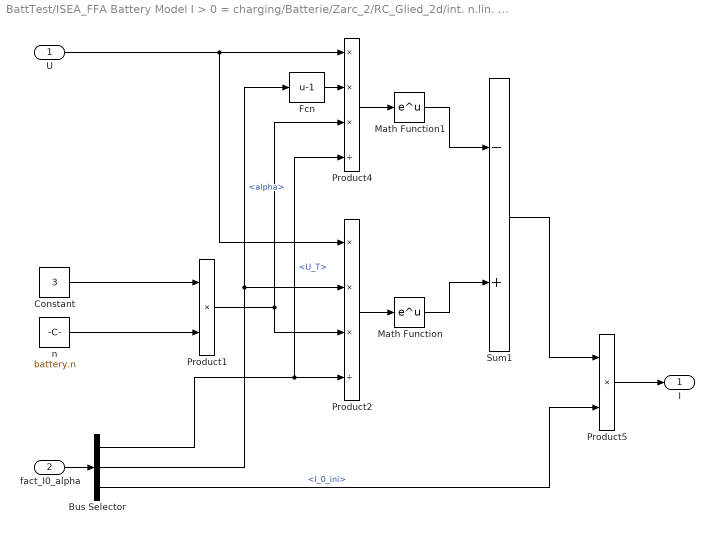
== system BattTest/ISEA_FFA Battery Model I > 0 = charging/Batterie/Zarc_2/RC_Glied_2d/int. n.lin. R2 ==
  U : Inport  Port=1  LatchInput=off
  fact_I0_alpha : Inport  Port=2  LatchInput=off
  Bus Selector : BusSelector  OutputSignals=U_T,alpha,I_0_ini  MuxedOutput=off
  Constant : Constant  Value=3
  Fcn : Fcn  Expr=u-1
  Math Function : Math  Operator=exp  OutputSignalType=auto
  Math Function1 : Math  Operator=exp  OutputSignalType=auto
  Product1 : Product  Inputs=**  Multiplication=Element-wise(.*)  SaturateOnIntegerOverflow=on
  Product2 : Product  Inputs=***/  Multiplication=Element-wise(.*)  SaturateOnIntegerOverflow=on
  Product4 : Product  Inputs=***/  Multiplication=Element-wise(.*)  SaturateOnIntegerOverflow=on
  Product5 : Product  Inputs=**  Multiplication=Element-wise(.*)  SaturateOnIntegerOverflow=on
  Sum1 : Sum  Inputs=-+  SaturateOnIntegerOverflow=on
  n : Constant  Value=battery.n
  I : Outport  Port=1
  wires:
  Constant/1 -> Product1/1
  Bus Selector/3 -> Product5/2  "<I_0_ini>"
  Product1/1 -> Product4/3, Product2/3
  n/1 -> Product1/2
  Product4/1 -> Math Function1/1
  Product5/1 -> I/1
  Sum1/1 -> Product5/1
  Math Function/1 -> Sum1/2
  Math Function1/1 -> Sum1/1
  Product2/1 -> Math Function/1
  U/1 -> Product2/1, Product4/1
  Fcn/1 -> Product4/2
  Bus Selector/2 -> Fcn/1, Product2/2  "<alpha>"
  Bus Selector/1 -> Product4/4, Product2/4  "<U_T>"
  fact_I0_alpha/1 -> Bus Selector/1
